simulink model "L4_2_lookup_table"  (R2025b)
settings: Solver=VariableStepAuto  StartTime=0.0  StopTime=4  MaxStep=0.01  RelTol=1e-3
settings Model: Creator=kimsteph  LastModifiedBy=kimsteph

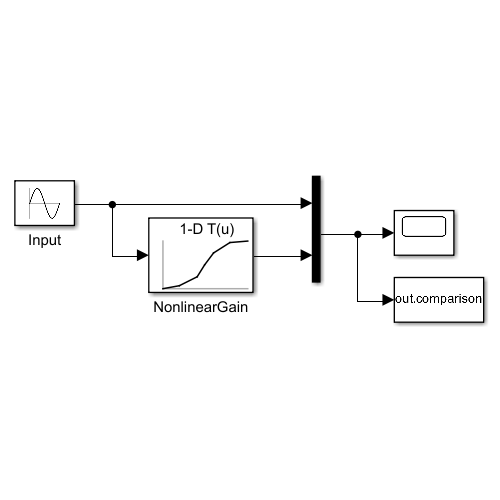
[thumbnail: Simulink's stored preview of the top-level diagram]
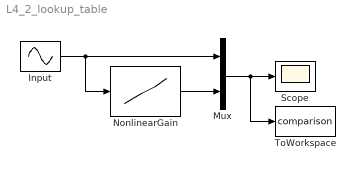
== system L4_2_lookup_table ==
  Input : Sin  Amplitude=5  Frequency=2*pi*0.5  SampleTime=0
  Mux : Mux  Inputs=2
  NonlinearGain : Lookup_n-D  NumberOfTableDimensions=1  BreakpointsForDimension1=[-5 -3 -1 0 1 3 5]  Table=[-1 -0.9 -0.5 0 0.5 0.9 1]  InternalRulePriority=Speed  RndMeth=Simplest
  Scope : Scope
  ToWorkspace : ToWorkspace  VariableName=comparison  SaveFormat=Timeseries  SampleTime=-1
  wires:
  Input/1 -> Mux/1, NonlinearGain/1
  NonlinearGain/1 -> Mux/2
  Mux/1 -> Scope/1, ToWorkspace/1
